simulink model "ECE314HW5_2c"  (R2017b)
settings: Solver=VariableStepAuto  StartTime=0.0  StopTime=10.0  RelTol=1e-3
values from neighbouring files (symbols this model uses):
  b = 20    [ECE314_HW4_1.m]    (also in ECE314_HW4_2.m = 2000; ECE314_HW4_2b.m = 200; ECE314_HW5_2c.m = 3769911.18431)
  c = fourier(b,a)    [ECE314_HW4_1.m]    (also in ECE314_HW4_2.m; ECE314_HW4_2b.m; ECE314_HW5_2c.m = 3.94784176044e+13)
  pw = 1e-9    (= 1e-09)    [ECE314_HW5_2c.m]
undefined symbols (not defined in the file or in its folder): amp, offset, per
settings Model: Creator=spenc  LastModifiedBy=spenc

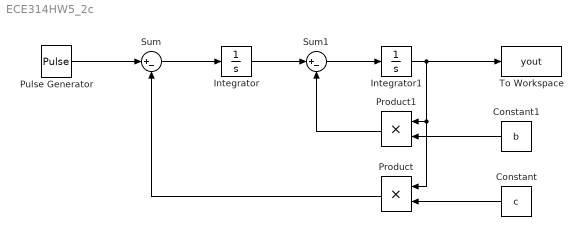
== system ECE314HW5_2c ==
  Constant : Constant  Value=c
  Constant1 : Constant  Value=b
  Integrator : Integrator
  Integrator1 : Integrator
  Product : Product
  Product1 : Product
  Pulse Generator : DiscretePulseGenerator  PulseType=Time based  Amplitude=amp  Period=per  PulseWidth=pw*100/per  PhaseDelay=offset
  Sum : Sum  Inputs=|+-
  Sum1 : Sum  Inputs=|+-
  To Workspace : ToWorkspace  VariableName=yout  SaveFormat=Timeseries  SampleTime=-1
  wires:
  Constant/1 -> Product/2
  Constant1/1 -> Product1/2
  Product1/1 -> Sum1/2
  Product/1 -> Sum/2
  Pulse Generator/1 -> Sum/1
  Sum/1 -> Integrator/1
  Integrator/1 -> Sum1/1
  Sum1/1 -> Integrator1/1
  Integrator1/1 -> To Workspace/1, Product/1, Product1/1
